simulink model "unitree_a1_base"  (R2022b)
settings: Solver=VariableStepAuto  StartTime=0.0  StopTime=5  FixedStep=0.005  RelTol=1e-3
values from neighbouring files (symbols this model uses):
  m = 12    [mpc.m]    (also in mpc_soln.m; qp_soln.m)
  N = 50    [mpc.m]    (also in mpc_caller.m = 20; qp_caller.m = params.N)
  X = [p; reshape(R, [9 1]); v; R'*w]    [mpc_caller.m]    (also in qp_caller.m)
undefined symbols (not defined in the file or in its folder): Y, Z
libraries: sm_lib x214, nesl_utility x113, simulink x1
(part 5 of 5)

== matlab function unitree_a1_base/MATLAB Function2 ==
  data: p input; R input; tau output; v input; p_hip input; p_foot input; v_foot input; q input; vd input; t input; pd_foot output; vd_foot output; pfinal_foot output; Fswing output; task input
function [tau, pd_foot, vd_foot, pfinal_foot, Fswing] = swing_controller(p, R, v, p_hip, p_foot, v_foot, q, vd, t, task)

pfinal_foot = zeros(12,1);

if task == 0 % standing
    [tau, pd_foot, vd_foot, Fswing] = foot_placement_standing(p, R, v, p_hip, p_foot, v_foot, q, t);
else % task == 1 % walking
    [tau, pd_foot, vd_foot, pfinal_foot, Fswing] = foot_placement_walking(p, R, v, p_hip, p_foot, v_foot, q, vd, t);
end


% select_leg = [0;0;1;0];
% tau = tau.*[select_leg;select_leg;select_leg;]

== matlab function unitree_a1_base/MATLAB Function3 ==
  data: p input; v input; w input; tau output; R input; q input; p1 input; p2 input; p3 input; p4 input; t input; F output
function [tau, F] = qp_controller_wrapper(p, v, w, R, q, p1, p2, p3, p4, t)
    [tau, F] = qp_caller(p, v, w, R, q, p1, p2, p3, p4, t);
end
